simulink model "CV_WLT_FM"  (R2020b)
settings: Solver=VariableStepAuto  StartTime=0.0  StopTime=inf  RelTol=1e-3
libraries: opclib x3, sldrtlib x1
settings Model: Creator=Ferdy  LastModifiedBy=Ferdy

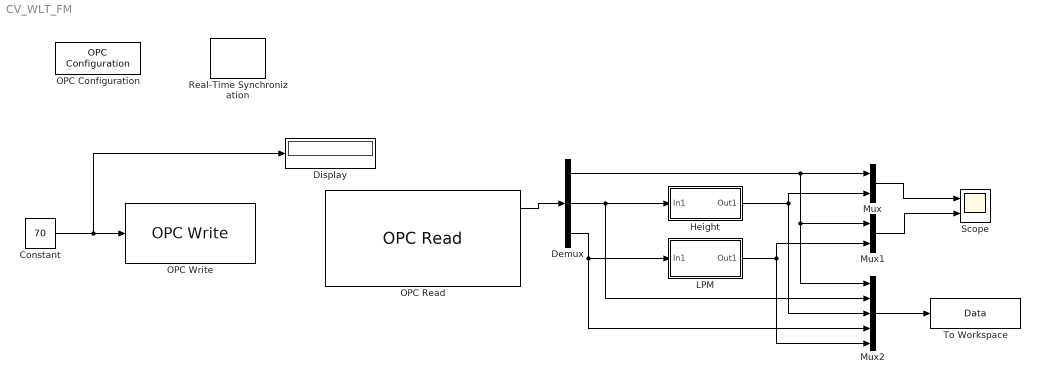
== system CV_WLT_FM ==
  Constant : Constant  Value=70
  Demux : Demux  Outputs=3
  Display : Display
  Height : Subsystem
  LPM : Subsystem
  Mux : Mux  Inputs=2
  Mux1 : Mux  Inputs=2
  Mux2 : Mux  Inputs=5
  OPC Configuration : opclib/OPC Configuration  opcServers=localhost/KEPware.KEPServerEx.V4/10  errMissingItems=Error  errReadWrite=Warn  errShutdown=Error  errRTViolation=Warn  rtEnable=on  speedup=1  showLatency=off  beingUsed=on
      settings: SourceProductBaseCode=OT
  OPC Read : opclib/OPC Read  serverHost=localhost  serverID=KEPware.KEPServerEx.V4  itemIDs=Fultek.CPU101F.ControlValve, Fultek.CPU101F.LVL, Fultek.CPU101F.InputFlow  readMode=Synchronous (cache)  dataType=double  updateRate=0.1  showQual=on  showTS=on  tsMode=Seconds since start
      settings: SourceProductBaseCode=OT
  OPC Write : opclib/OPC Write  serverHost=localhost  serverID=KEPware.KEPServerEx.V4  itemIDs=Fultek.CPU101F.ControlValve  writeMode=Synchronous  updateRate=0
      settings: SourceProductBaseCode=OT
  Real-Time Synchronization : sldrtlib/Real-Time Synchronization  SampleTime=0.1  MaxMissedTicks=10  ShowMissedTicks=off  YieldWhenWaiting=off
  Scope : Scope  NumInputPorts=2
  To Workspace : ToWorkspace  VariableName=Data  SaveFormat=Timeseries  SampleTime=-1
  wires:
  Constant/1 -> OPC Write/1, Display/1
  Mux/1 -> Scope/1
  Mux1/1 -> Scope/2
  Mux2/1 -> To Workspace/1
  OPC Read/1 -> Demux/1
  Demux/1 -> Mux/1, Mux2/1, Mux1/1
  Demux/2 -> Mux2/2, Height/1(In1)
  Demux/3 -> Mux2/4, LPM/1(In1)
  Height/1(Out1) -> Mux2/3, Mux/2
  LPM/1(Out1) -> Mux1/2, Mux2/5

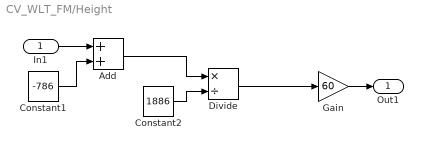
== system CV_WLT_FM/Height ==
  In1 : Inport
  Add : Sum
  Constant1 : Constant  Value=-786
  Constant2 : Constant  Value=1886
  Divide : Product  Inputs=*/
  Gain : Gain  Gain=60
  Out1 : Outport
  wires:
  Add/1 -> Divide/1
  Divide/1 -> Gain/1
  Constant1/1 -> Add/2
  Constant2/1 -> Divide/2
  In1/1 -> Add/1
  Gain/1 -> Out1/1

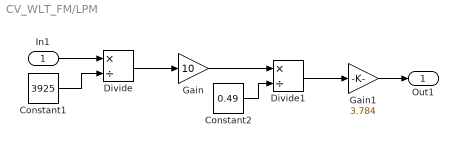
== system CV_WLT_FM/LPM ==
  In1 : Inport
  Constant1 : Constant  Value=3925
  Constant2 : Constant  Value=0.49
  Divide : Product  Inputs=*/
  Divide1 : Product  Inputs=*/
  Gain : Gain  Gain=10
  Gain1 : Gain  Gain=3.784
  Out1 : Outport
  wires:
  Divide/1 -> Gain/1
  Constant1/1 -> Divide/2
  Constant2/1 -> Divide1/2
  Gain/1 -> Divide1/1
  Divide1/1 -> Gain1/1
  In1/1 -> Divide/1
  Gain1/1 -> Out1/1
